simulink model "HANcoder_E407_TTA_Controller_v4_7"  (R2018b)
settings: Solver=FixedStepDiscrete  StartTime=0.0  StopTime=1  FixedStep=0.01  RelTol=1e-3
PreLoadFcn:
  | librarySetup
  | eval([bdroot,'_startup']) %Calling [modelName]_startup.m
values from neighbouring files (symbols this model uses):
  Backup_Board = 0    [HANcoder_E407_TTA_Controller_v3_5_startup.m]    (also in HANcoder_E407_TTA_Controller_v4_6_startup.m; HANcoder_E407_TTA_Controller_v4_7_startup.m; HANcoder_E407_TTA_Controller_v4_startup.m)
  basic_cycle_duration_bc0 = TM_Reset_Board   + COMP_duration    (= 212)    [HANcoder_E407_TTA_Controller_v3_5_startup.m]    (also in HANcoder_E407_TTA_Controller_v4_6_startup.m; HANcoder_E407_TTA_Controller_v4_7_startup.m; HANcoder_E407_TTA_Controller_v4_startup.m)
  basic_cycle_duration_bc1 = TM_Reset_Var_bc1 + COMP_duration    (= 288)    [HANcoder_E407_TTA_Controller_v3_5_startup.m]    (also in HANcoder_E407_TTA_Controller_v4_6_startup.m = 332; HANcoder_E407_TTA_Controller_v4_7_startup.m = 372; HANcoder_E407_TTA_Controller_v4_startup.m = 332)
  comm_delay_estimation1 = round(comm_delay_measured1*hardware_granularity/frequency_IRQ)    [HANcoder_E407_TTA_Controller_v3_5_startup.m]    (also in HANcoder_E407_TTA_Controller_v4_6_startup.m; HANcoder_E407_TTA_Controller_v4_7_startup.m; HANcoder_E407_TTA_Controller_v4_startup.m)
  comm_delay_estimation2 = round(comm_delay_measured2*hardware_granularity/frequency_IRQ)    [HANcoder_E407_TTA_Controller_v3_5_startup.m]    (also in HANcoder_E407_TTA_Controller_v4_6_startup.m; HANcoder_E407_TTA_Controller_v4_7_startup.m; HANcoder_E407_TTA_Controller_v4_startup.m)
  COMM_Period = 40    [HANcoder_E407_TTA_Controller_v3_5_startup.m]    (also in HANcoder_E407_TTA_Controller_v4_6_startup.m; HANcoder_E407_TTA_Controller_v4_7_startup.m; HANcoder_E407_TTA_Controller_v4_startup.m)
  COMM_Phase1 = Simulink.Parameter    [HANcoder_E407_TTA_Controller_v3_5_startup.m]    (also in HANcoder_E407_TTA_Controller_v4_6_startup.m; HANcoder_E407_TTA_Controller_v4_7_startup.m; HANcoder_E407_TTA_Controller_v4_startup.m)
  COMM_Phase2 = Simulink.Parameter    [HANcoder_E407_TTA_Controller_v3_5_startup.m]    (also in HANcoder_E407_TTA_Controller_v4_6_startup.m; HANcoder_E407_TTA_Controller_v4_7_startup.m; HANcoder_E407_TTA_Controller_v4_startup.m)
  COMM_Phase_init1 = Simulink.Parameter    [HANcoder_E407_TTA_Controller_v3_5_startup.m]    (also in HANcoder_E407_TTA_Controller_v4_6_startup.m; HANcoder_E407_TTA_Controller_v4_7_startup.m; HANcoder_E407_TTA_Controller_v4_startup.m)
  COMM_Phase_init2 = Simulink.Parameter    [HANcoder_E407_TTA_Controller_v3_5_startup.m]    (also in HANcoder_E407_TTA_Controller_v4_6_startup.m; HANcoder_E407_TTA_Controller_v4_7_startup.m; HANcoder_E407_TTA_Controller_v4_startup.m)
  COMP_duration = 4    [HANcoder_E407_TTA_Controller_v3_5_startup.m]    (also in HANcoder_E407_TTA_Controller_v4_6_startup.m; HANcoder_E407_TTA_Controller_v4_7_startup.m; HANcoder_E407_TTA_Controller_v4_startup.m)
  Controller1_Board = 1    [HANcoder_E407_TTA_Controller_v3_5_startup.m]    (also in HANcoder_E407_TTA_Controller_v4_6_startup.m; HANcoder_E407_TTA_Controller_v4_7_startup.m; HANcoder_E407_TTA_Controller_v4_startup.m)
  Controller2_Board = 2    [HANcoder_E407_TTA_Controller_v3_5_startup.m]    (also in HANcoder_E407_TTA_Controller_v4_6_startup.m; HANcoder_E407_TTA_Controller_v4_7_startup.m; HANcoder_E407_TTA_Controller_v4_startup.m)
  Controller3_Board = 3    [HANcoder_E407_TTA_Controller_v3_5_startup.m]    (also in HANcoder_E407_TTA_Controller_v4_6_startup.m; HANcoder_E407_TTA_Controller_v4_7_startup.m; HANcoder_E407_TTA_Controller_v4_startup.m)
  delta_a_set = Simulink.Parameter    [HANcoder_E407_TTA_Controller_v3_5_startup.m]    (also in HANcoder_E407_TTA_Controller_v4_6_startup.m; HANcoder_E407_TTA_Controller_v4_7_startup.m; HANcoder_E407_TTA_Controller_v4_startup.m)
  delta_f_set = Simulink.Parameter    [HANcoder_E407_TTA_Controller_v3_5_startup.m]    (also in HANcoder_E407_TTA_Controller_v4_6_startup.m; HANcoder_E407_TTA_Controller_v4_7_startup.m; HANcoder_E407_TTA_Controller_v4_startup.m)
  delta_max = 1    [HANcoder_E407_TTA_Controller_v3_5_startup.m]    (also in HANcoder_E407_TTA_Controller_v4_6_startup.m; HANcoder_E407_TTA_Controller_v4_7_startup.m; HANcoder_E407_TTA_Controller_v4_startup.m)
  delta_min = -1    [HANcoder_E407_TTA_Controller_v3_5_startup.m]    (also in HANcoder_E407_TTA_Controller_v4_6_startup.m; HANcoder_E407_TTA_Controller_v4_7_startup.m; HANcoder_E407_TTA_Controller_v4_startup.m)
  delta_precision = 6    [HANcoder_E407_TTA_Controller_v3_5_startup.m]    (also in HANcoder_E407_TTA_Controller_v4_6_startup.m; HANcoder_E407_TTA_Controller_v4_7_startup.m; HANcoder_E407_TTA_Controller_v4_startup.m)
  e_width = 0.1    [HANcoder_E407_TTA_Controller_v3_5_startup.m]    (also in HANcoder_E407_TTA_Controller_v4_6_startup.m; HANcoder_E407_TTA_Controller_v4_7_startup.m; HANcoder_E407_TTA_Controller_v4_startup.m)
  frequency_IRQ = 100    [HANcoder_E407_2xCAN_TEST_startup.m]    (also in HANcoder_E407_TTA_Controller_v3_5_startup.m; HANcoder_E407_TTA_Controller_v4_6_startup.m; HANcoder_E407_TTA_Controller_v4_7_startup.m; HANcoder_E407_TTA_Controller_v4_startup.m)
  HANtuneOverride = Simulink.Parameter    [HANcoder_E407_2xCAN_TEST_startup.m]    (also in HANcoder_E407_TTA_Controller_v3_5_startup.m; HANcoder_E407_TTA_Controller_v4_6_startup.m; HANcoder_E407_TTA_Controller_v4_7_startup.m; HANcoder_E407_TTA_Controller_v4_startup.m)
  hardware_granularity = 1000000    [HANcoder_E407_2xCAN_TEST_startup.m]    (also in HANcoder_E407_TTA_Controller_v3_5_startup.m; HANcoder_E407_TTA_Controller_v4_6_startup.m; HANcoder_E407_TTA_Controller_v4_7_startup.m; HANcoder_E407_TTA_Controller_v4_startup.m)
  I_a = 2.25    [HANcoder_E407_TTA_Controller_v3_5_startup.m]    (also in HANcoder_E407_TTA_Controller_v4_6_startup.m; HANcoder_E407_TTA_Controller_v4_7_startup.m; HANcoder_E407_TTA_Controller_v4_startup.m)
  I_f = 2.25    [HANcoder_E407_TTA_Controller_v3_5_startup.m]    (also in HANcoder_E407_TTA_Controller_v4_6_startup.m; HANcoder_E407_TTA_Controller_v4_7_startup.m; HANcoder_E407_TTA_Controller_v4_startup.m)
  idle_time_init = basic_cycle_duration_bc0 + basic_cycle_duration_bc1    (= 500)    [HANcoder_E407_TTA_Controller_v3_5_startup.m]    (also in HANcoder_E407_TTA_Controller_v4_6_startup.m = 544; HANcoder_E407_TTA_Controller_v4_7_startup.m = 584; HANcoder_E407_TTA_Controller_v4_startup.m = 544)
  Input_Gen_Board = 4    [HANcoder_E407_TTA_Controller_v3_5_startup.m]    (also in HANcoder_E407_TTA_Controller_v4_6_startup.m; HANcoder_E407_TTA_Controller_v4_7_startup.m; HANcoder_E407_TTA_Controller_v4_startup.m)
  LA_Clock_Gr = 1    [HANcoder_E407_TTA_Controller_v3_5_startup.m]    (also in HANcoder_E407_TTA_Controller_v4_6_startup.m; HANcoder_E407_TTA_Controller_v4_7_startup.m; HANcoder_E407_TTA_Controller_v4_startup.m)
  LA_COMM_dly = 1    [HANcoder_E407_TTA_Controller_v3_5_startup.m]    (also in HANcoder_E407_TTA_Controller_v4_6_startup.m; HANcoder_E407_TTA_Controller_v4_7_startup.m; HANcoder_E407_TTA_Controller_v4_startup.m)
  LA_COMM_Err = 1    [HANcoder_E407_TTA_Controller_v3_5_startup.m]    (also in HANcoder_E407_TTA_Controller_v4_6_startup.m; HANcoder_E407_TTA_Controller_v4_7_startup.m; HANcoder_E407_TTA_Controller_v4_startup.m)
  LA_E_Desync = 1    [HANcoder_E407_TTA_Controller_v3_5_startup.m]    (also in HANcoder_E407_TTA_Controller_v4_6_startup.m; HANcoder_E407_TTA_Controller_v4_7_startup.m; HANcoder_E407_TTA_Controller_v4_startup.m)
  LA_MEX_Flag = 1    [HANcoder_E407_TTA_Controller_v3_5_startup.m]    (also in HANcoder_E407_TTA_Controller_v4_6_startup.m; HANcoder_E407_TTA_Controller_v4_7_startup.m; HANcoder_E407_TTA_Controller_v4_startup.m)
  LA_Task_Act = 1    [HANcoder_E407_TTA_Controller_v3_5_startup.m]    (also in HANcoder_E407_TTA_Controller_v4_6_startup.m; HANcoder_E407_TTA_Controller_v4_7_startup.m; HANcoder_E407_TTA_Controller_v4_startup.m)
  m_v = 100.0    (= 100)    [HANcoder_E407_TTA_Controller_v3_5_startup.m]    (also in HANcoder_E407_TTA_Controller_v4_6_startup.m; HANcoder_E407_TTA_Controller_v4_7_startup.m; HANcoder_E407_TTA_Controller_v4_startup.m)
  Master_Role = 1    [HANcoder_E407_TTA_Controller_v3_5_startup.m]    (also in HANcoder_E407_TTA_Controller_v4_6_startup.m; HANcoder_E407_TTA_Controller_v4_7_startup.m; HANcoder_E407_TTA_Controller_v4_startup.m)
  matrix_cycle_duration = basic_cycle_duration_bc0 + basic_cycle_duration_bc1    (= 500)    [HANcoder_E407_TTA_Controller_v3_5_startup.m]    (also in HANcoder_E407_TTA_Controller_v4_6_startup.m = 544; HANcoder_E407_TTA_Controller_v4_7_startup.m = 584; HANcoder_E407_TTA_Controller_v4_startup.m = 544)
  matrix_rows = 2    [HANcoder_E407_TTA_Controller_v3_5_startup.m]    (also in HANcoder_E407_TTA_Controller_v4_6_startup.m; HANcoder_E407_TTA_Controller_v4_7_startup.m; HANcoder_E407_TTA_Controller_v4_startup.m)
  max_desync = 15    [HANcoder_E407_TTA_Controller_v3_5_startup.m]    (also in HANcoder_E407_TTA_Controller_v4_6_startup.m; HANcoder_E407_TTA_Controller_v4_7_startup.m = 30; HANcoder_E407_TTA_Controller_v4_startup.m)
  max_num_msgs_CAN1 = 2^Tx_bit_number-1    (= 7)    [HANcoder_E407_TTA_Controller_v3_5_startup.m]    (also in HANcoder_E407_TTA_Controller_v4_6_startup.m = 15; HANcoder_E407_TTA_Controller_v4_7_startup.m = 15; HANcoder_E407_TTA_Controller_v4_startup.m)
  max_num_msgs_CAN2 = max_num_msgs_CAN1    (= 7)    [HANcoder_E407_TTA_Controller_v3_5_startup.m]    (also in HANcoder_E407_TTA_Controller_v4_6_startup.m = 15; HANcoder_E407_TTA_Controller_v4_7_startup.m = 15; HANcoder_E407_TTA_Controller_v4_startup.m)
  min_desync = (-1)*max_desync    (= -15)    [HANcoder_E407_TTA_Controller_v3_5_startup.m]    (also in HANcoder_E407_TTA_Controller_v4_6_startup.m; HANcoder_E407_TTA_Controller_v4_7_startup.m = -30; HANcoder_E407_TTA_Controller_v4_startup.m)
  OutControl1_ID = 23    [HANcoder_E407_TTA_Controller_v3_5_startup.m]    (also in HANcoder_E407_TTA_Controller_v4_6_startup.m; HANcoder_E407_TTA_Controller_v4_7_startup.m; HANcoder_E407_TTA_Controller_v4_startup.m)
  OutControl2_ID = 24    [HANcoder_E407_TTA_Controller_v3_5_startup.m]    (also in HANcoder_E407_TTA_Controller_v4_6_startup.m; HANcoder_E407_TTA_Controller_v4_7_startup.m; HANcoder_E407_TTA_Controller_v4_startup.m)
  OutEmulator_ID = 25    [HANcoder_E407_TTA_Controller_v3_5_startup.m]    (also in HANcoder_E407_TTA_Controller_v4_6_startup.m = 26; HANcoder_E407_TTA_Controller_v4_7_startup.m = 26; HANcoder_E407_TTA_Controller_v4_startup.m)
  OutMaster_ID = 25    [HANcoder_E407_TTA_Controller_v4_6_startup.m]    (also in HANcoder_E407_TTA_Controller_v4_7_startup.m; HANcoder_E407_TTA_Controller_v4_startup.m = 26)
  R_al = 0.10    (= 0.1)    [HANcoder_E407_TTA_Controller_v3_5_startup.m]    (also in HANcoder_E407_TTA_Controller_v4_6_startup.m; HANcoder_E407_TTA_Controller_v4_7_startup.m; HANcoder_E407_TTA_Controller_v4_startup.m)
  R_ar = 0.10    (= 0.1)    [HANcoder_E407_TTA_Controller_v3_5_startup.m]    (also in HANcoder_E407_TTA_Controller_v4_6_startup.m; HANcoder_E407_TTA_Controller_v4_7_startup.m; HANcoder_E407_TTA_Controller_v4_startup.m)
  R_fl = 0.10    (= 0.1)    [HANcoder_E407_TTA_Controller_v3_5_startup.m]    (also in HANcoder_E407_TTA_Controller_v4_6_startup.m; HANcoder_E407_TTA_Controller_v4_7_startup.m; HANcoder_E407_TTA_Controller_v4_startup.m)
  R_fr = 0.10    (= 0.1)    [HANcoder_E407_TTA_Controller_v3_5_startup.m]    (also in HANcoder_E407_TTA_Controller_v4_6_startup.m; HANcoder_E407_TTA_Controller_v4_7_startup.m; HANcoder_E407_TTA_Controller_v4_startup.m)
  script_run = Simulink.Parameter    [HANcoder_E407_TTA_Controller_v3_5_startup.m]    (also in HANcoder_E407_TTA_Controller_v4_6_startup.m; HANcoder_E407_TTA_Controller_v4_7_startup.m; HANcoder_E407_TTA_Controller_v4_startup.m)
  SensorValues_ID = 22    [HANcoder_E407_TTA_Controller_v3_5_startup.m]    (also in HANcoder_E407_TTA_Controller_v4_6_startup.m; HANcoder_E407_TTA_Controller_v4_7_startup.m; HANcoder_E407_TTA_Controller_v4_startup.m)
  SetValues_ID = 21    [HANcoder_E407_TTA_Controller_v3_5_startup.m]    (also in HANcoder_E407_TTA_Controller_v4_6_startup.m; HANcoder_E407_TTA_Controller_v4_7_startup.m; HANcoder_E407_TTA_Controller_v4_startup.m)
  Slave_Role = 2    [HANcoder_E407_TTA_Controller_v3_5_startup.m]    (also in HANcoder_E407_TTA_Controller_v4_6_startup.m; HANcoder_E407_TTA_Controller_v4_7_startup.m; HANcoder_E407_TTA_Controller_v4_startup.m)
  speed_k_d = Simulink.Parameter    [HANcoder_E407_TTA_Controller_v3_5_startup.m]    (also in HANcoder_E407_TTA_Controller_v4_6_startup.m; HANcoder_E407_TTA_Controller_v4_7_startup.m; HANcoder_E407_TTA_Controller_v4_startup.m)
  speed_k_i = Simulink.Parameter    [HANcoder_E407_TTA_Controller_v3_5_startup.m]    (also in HANcoder_E407_TTA_Controller_v4_6_startup.m; HANcoder_E407_TTA_Controller_v4_7_startup.m; HANcoder_E407_TTA_Controller_v4_startup.m)
  speed_k_p = Simulink.Parameter    [HANcoder_E407_TTA_Controller_v3_5_startup.m]    (also in HANcoder_E407_TTA_Controller_v4_6_startup.m; HANcoder_E407_TTA_Controller_v4_7_startup.m; HANcoder_E407_TTA_Controller_v4_startup.m)
  speed_max = 10    [HANcoder_E407_TTA_Controller_v3_5_startup.m]    (also in HANcoder_E407_TTA_Controller_v4_6_startup.m; HANcoder_E407_TTA_Controller_v4_7_startup.m; HANcoder_E407_TTA_Controller_v4_startup.m)
  speed_min = -10    [HANcoder_E407_TTA_Controller_v3_5_startup.m]    (also in HANcoder_E407_TTA_Controller_v4_6_startup.m; HANcoder_E407_TTA_Controller_v4_7_startup.m; HANcoder_E407_TTA_Controller_v4_startup.m)
  speed_precision = 3    [HANcoder_E407_TTA_Controller_v3_5_startup.m]    (also in HANcoder_E407_TTA_Controller_v4_6_startup.m; HANcoder_E407_TTA_Controller_v4_7_startup.m; HANcoder_E407_TTA_Controller_v4_startup.m)
  Sync_ID = 1    [HANcoder_E407_TTA_Controller_v3_5_startup.m]    (also in HANcoder_E407_TTA_Controller_v4_6_startup.m; HANcoder_E407_TTA_Controller_v4_7_startup.m; HANcoder_E407_TTA_Controller_v4_startup.m)
  tau_max = 5    [HANcoder_E407_TTA_Controller_v3_5_startup.m]    (also in HANcoder_E407_TTA_Controller_v4_6_startup.m; HANcoder_E407_TTA_Controller_v4_7_startup.m; HANcoder_E407_TTA_Controller_v4_startup.m)
  tau_min = -5    [HANcoder_E407_TTA_Controller_v3_5_startup.m]    (also in HANcoder_E407_TTA_Controller_v4_6_startup.m; HANcoder_E407_TTA_Controller_v4_7_startup.m; HANcoder_E407_TTA_Controller_v4_startup.m)
  tau_range = abs(tau_max) + abs(tau_min)    [HANcoder_E407_TTA_Controller_v3_5_startup.m]    (also in HANcoder_E407_TTA_Controller_v4_6_startup.m; HANcoder_E407_TTA_Controller_v4_7_startup.m; HANcoder_E407_TTA_Controller_v4_startup.m)
  theta_max = (speed_max/R_fr)*matrix_cycle_duration*frequency_IRQ/hardware_granularity    (= 5)    [HANcoder_E407_TTA_Controller_v3_5_startup.m]    (also in HANcoder_E407_TTA_Controller_v4_6_startup.m = 5.44; HANcoder_E407_TTA_Controller_v4_7_startup.m = 5.84; HANcoder_E407_TTA_Controller_v4_startup.m = 5.44)
  theta_min = (-1)*theta_max    (= -5)    [HANcoder_E407_TTA_Controller_v3_5_startup.m]    (also in HANcoder_E407_TTA_Controller_v4_6_startup.m = -5.44; HANcoder_E407_TTA_Controller_v4_7_startup.m = -5.84; HANcoder_E407_TTA_Controller_v4_startup.m = -5.44)
  theta_precision = 7-(fix(log2(theta_max))+1)    [HANcoder_E407_TTA_Controller_v3_5_startup.m]    (also in HANcoder_E407_TTA_Controller_v4_6_startup.m; HANcoder_E407_TTA_Controller_v4_7_startup.m; HANcoder_E407_TTA_Controller_v4_startup.m)
  Tl_a = 0.6    [HANcoder_E407_TTA_Controller_v3_5_startup.m]    (also in HANcoder_E407_TTA_Controller_v4_6_startup.m; HANcoder_E407_TTA_Controller_v4_7_startup.m; HANcoder_E407_TTA_Controller_v4_startup.m)
  Tl_f = 0.6    [HANcoder_E407_TTA_Controller_v3_5_startup.m]    (also in HANcoder_E407_TTA_Controller_v4_6_startup.m; HANcoder_E407_TTA_Controller_v4_7_startup.m; HANcoder_E407_TTA_Controller_v4_startup.m)
  TM_Check_Output_Control1 = TM_COMM_Output_Control1 + COMM_duration    (= 188)    [HANcoder_E407_TTA_Controller_v3_5_startup.m]    (also in HANcoder_E407_TTA_Controller_v4_6_startup.m; HANcoder_E407_TTA_Controller_v4_7_startup.m; HANcoder_E407_TTA_Controller_v4_startup.m)
  TM_Check_Output_Control2 = TM_COMM_Output_Control2 + COMM_duration    (= 232)    [HANcoder_E407_TTA_Controller_v3_5_startup.m]    (also in HANcoder_E407_TTA_Controller_v4_6_startup.m; HANcoder_E407_TTA_Controller_v4_7_startup.m; HANcoder_E407_TTA_Controller_v4_startup.m)
  TM_Check_Output_Emulator = TM_COMM_Output_Emulator + COMM_duration    (= 280)    [HANcoder_E407_TTA_Controller_v3_5_startup.m]    (also in HANcoder_E407_TTA_Controller_v4_6_startup.m = 320; HANcoder_E407_TTA_Controller_v4_7_startup.m = 360; HANcoder_E407_TTA_Controller_v4_startup.m = 320)
  TM_Check_Output_Emulator_2 = TM_Check_Output_Emulator + 2    (= 282)    [HANcoder_E407_TTA_Controller_v3_5_startup.m]    (also in HANcoder_E407_TTA_Controller_v4_6_startup.m = 322; HANcoder_E407_TTA_Controller_v4_7_startup.m = 362; HANcoder_E407_TTA_Controller_v4_startup.m = 322)
  TM_Check_Output_Emulator_3 = TM_Check_Output_Emulator_2 + 2    (= 324)    [HANcoder_E407_TTA_Controller_v4_6_startup.m]    (also in HANcoder_E407_TTA_Controller_v4_7_startup.m = 364; HANcoder_E407_TTA_Controller_v4_startup.m)
  TM_Check_Output_Master = TM_COMM_Output_Master + COMM_duration    (= 312)    [HANcoder_E407_TTA_Controller_v4_7_startup.m]
  TM_Check_Sensor_Values = TM_COMM_Sensor_Values + COMM_duration    (= 132)    [HANcoder_E407_TTA_Controller_v3_5_startup.m]    (also in HANcoder_E407_TTA_Controller_v4_6_startup.m; HANcoder_E407_TTA_Controller_v4_7_startup.m; HANcoder_E407_TTA_Controller_v4_startup.m)
  TM_Check_Sensor_Values_2 = TM_Check_Sensor_Values + 2    (= 134)    [HANcoder_E407_TTA_Controller_v3_5_startup.m]    (also in HANcoder_E407_TTA_Controller_v4_6_startup.m; HANcoder_E407_TTA_Controller_v4_7_startup.m; HANcoder_E407_TTA_Controller_v4_startup.m)
  TM_Check_Set_Values = TM_COMM_Set_Values + COMM_duration    (= 88)    [HANcoder_E407_TTA_Controller_v3_5_startup.m]    (also in HANcoder_E407_TTA_Controller_v4_6_startup.m; HANcoder_E407_TTA_Controller_v4_7_startup.m; HANcoder_E407_TTA_Controller_v4_startup.m)
  TM_Check_Set_Values_2 = TM_Check_Set_Values + 2    (= 90)    [HANcoder_E407_TTA_Controller_v3_5_startup.m]    (also in HANcoder_E407_TTA_Controller_v4_6_startup.m; HANcoder_E407_TTA_Controller_v4_7_startup.m; HANcoder_E407_TTA_Controller_v4_startup.m)
  TM_Check_Sync = TM_COMM_Sync   + COMM_duration    (= 40)    [HANcoder_E407_TTA_Controller_v3_5_startup.m]    (also in HANcoder_E407_TTA_Controller_v4_6_startup.m; HANcoder_E407_TTA_Controller_v4_7_startup.m; HANcoder_E407_TTA_Controller_v4_startup.m)
  TM_Check_TOuts = TM_Count_Vote3 + COMP_duration    (= 196)    [HANcoder_E407_TTA_Controller_v3_5_startup.m]    (also in HANcoder_E407_TTA_Controller_v4_6_startup.m; HANcoder_E407_TTA_Controller_v4_7_startup.m; HANcoder_E407_TTA_Controller_v4_startup.m)
  TM_Check_Vote1 = TM_COMM_Vote1  + COMM_duration    (= 92)    [HANcoder_E407_TTA_Controller_v3_5_startup.m]    (also in HANcoder_E407_TTA_Controller_v4_6_startup.m; HANcoder_E407_TTA_Controller_v4_7_startup.m; HANcoder_E407_TTA_Controller_v4_startup.m)
  TM_Check_Vote2 = TM_COMM_Vote2  + COMM_duration    (= 140)    [HANcoder_E407_TTA_Controller_v3_5_startup.m]    (also in HANcoder_E407_TTA_Controller_v4_6_startup.m; HANcoder_E407_TTA_Controller_v4_7_startup.m; HANcoder_E407_TTA_Controller_v4_startup.m)
  TM_Check_Vote2_2 = TM_Check_Vote2 + 2    (= 142)    [HANcoder_E407_TTA_Controller_v3_5_startup.m]    (also in HANcoder_E407_TTA_Controller_v4_6_startup.m; HANcoder_E407_TTA_Controller_v4_7_startup.m; HANcoder_E407_TTA_Controller_v4_startup.m)
  TM_Check_Vote3 = TM_COMM_Vote3  + COMM_duration    (= 188)    [HANcoder_E407_TTA_Controller_v3_5_startup.m]    (also in HANcoder_E407_TTA_Controller_v4_6_startup.m; HANcoder_E407_TTA_Controller_v4_7_startup.m; HANcoder_E407_TTA_Controller_v4_startup.m)
  TM_COMM_Output_Control1 = TM_Velocity + COMP_duration    (= 148)    [HANcoder_E407_TTA_Controller_v3_5_startup.m]    (also in HANcoder_E407_TTA_Controller_v4_6_startup.m; HANcoder_E407_TTA_Controller_v4_7_startup.m; HANcoder_E407_TTA_Controller_v4_startup.m)
  TM_COMM_Output_Control2 = TM_Check_Output_Control1 + COMP_duration    (= 192)    [HANcoder_E407_TTA_Controller_v3_5_startup.m]    (also in HANcoder_E407_TTA_Controller_v4_6_startup.m; HANcoder_E407_TTA_Controller_v4_7_startup.m; HANcoder_E407_TTA_Controller_v4_startup.m)
  TM_COMM_Output_Emulator = TM_TMR + COMP_duration    (= 240)    [HANcoder_E407_TTA_Controller_v3_5_startup.m]    (also in HANcoder_E407_TTA_Controller_v4_6_startup.m = 280; HANcoder_E407_TTA_Controller_v4_7_startup.m = 320; HANcoder_E407_TTA_Controller_v4_startup.m = 280)
  TM_COMM_Output_Master = TM_Check_Output_Control2 + COMM_duration    (= 272)    [HANcoder_E407_TTA_Controller_v4_6_startup.m]    (also in HANcoder_E407_TTA_Controller_v4_7_startup.m; HANcoder_E407_TTA_Controller_v4_startup.m)
  TM_COMM_Sensor_Values = TM_Check_Set_Values + COMP_duration    (= 92)    [HANcoder_E407_TTA_Controller_v3_5_startup.m]    (also in HANcoder_E407_TTA_Controller_v4_6_startup.m; HANcoder_E407_TTA_Controller_v4_7_startup.m; HANcoder_E407_TTA_Controller_v4_startup.m)
  TM_COMM_Set_Values = TM_Update_LT + COMP_duration    (= 48)    [HANcoder_E407_TTA_Controller_v3_5_startup.m]    (also in HANcoder_E407_TTA_Controller_v4_6_startup.m; HANcoder_E407_TTA_Controller_v4_7_startup.m; HANcoder_E407_TTA_Controller_v4_startup.m)
  TM_COMM_Sync = basic_cycle_start    (= 0)    [HANcoder_E407_TTA_Controller_v3_5_startup.m]    (also in HANcoder_E407_TTA_Controller_v4_6_startup.m; HANcoder_E407_TTA_Controller_v4_7_startup.m; HANcoder_E407_TTA_Controller_v4_startup.m)
  TM_COMM_Vote1 = TM_Vote_Dec    + COMP_duration    (= 52)    [HANcoder_E407_TTA_Controller_v3_5_startup.m]    (also in HANcoder_E407_TTA_Controller_v4_6_startup.m; HANcoder_E407_TTA_Controller_v4_7_startup.m; HANcoder_E407_TTA_Controller_v4_startup.m)
  TM_COMM_Vote2 = TM_Count_Vote1 + COMP_duration    (= 100)    [HANcoder_E407_TTA_Controller_v3_5_startup.m]    (also in HANcoder_E407_TTA_Controller_v4_6_startup.m; HANcoder_E407_TTA_Controller_v4_7_startup.m; HANcoder_E407_TTA_Controller_v4_startup.m)
  TM_COMM_Vote3 = TM_Count_Vote2 + COMP_duration    (= 148)    [HANcoder_E407_TTA_Controller_v3_5_startup.m]    (also in HANcoder_E407_TTA_Controller_v4_6_startup.m; HANcoder_E407_TTA_Controller_v4_7_startup.m; HANcoder_E407_TTA_Controller_v4_startup.m)
  TM_Count_Vote1 = TM_Check_Vote1 + COMP_duration    (= 96)    [HANcoder_E407_TTA_Controller_v3_5_startup.m]    (also in HANcoder_E407_TTA_Controller_v4_6_startup.m; HANcoder_E407_TTA_Controller_v4_7_startup.m; HANcoder_E407_TTA_Controller_v4_startup.m)
  TM_Count_Vote2 = TM_Check_Vote2 + COMP_duration    (= 144)    [HANcoder_E407_TTA_Controller_v3_5_startup.m]    (also in HANcoder_E407_TTA_Controller_v4_6_startup.m; HANcoder_E407_TTA_Controller_v4_7_startup.m; HANcoder_E407_TTA_Controller_v4_startup.m)
  TM_Count_Vote3 = TM_Check_Vote3 + COMP_duration    (= 192)    [HANcoder_E407_TTA_Controller_v3_5_startup.m]    (also in HANcoder_E407_TTA_Controller_v4_6_startup.m; HANcoder_E407_TTA_Controller_v4_7_startup.m; HANcoder_E407_TTA_Controller_v4_startup.m)
  TM_Data_bc0 = TM_COMM_Sync    (= 0)    [HANcoder_E407_TTA_Controller_v3_5_startup.m]    (also in HANcoder_E407_TTA_Controller_v4_6_startup.m; HANcoder_E407_TTA_Controller_v4_7_startup.m; HANcoder_E407_TTA_Controller_v4_startup.m)
  TM_Data_bc1 = TM_Data_bc0(1:4)    [HANcoder_E407_TTA_Controller_v3_5_startup.m]    (also in HANcoder_E407_TTA_Controller_v4_6_startup.m; HANcoder_E407_TTA_Controller_v4_7_startup.m; HANcoder_E407_TTA_Controller_v4_startup.m)
  TM_New_Master = TM_Check_TOuts + COMP_duration    (= 200)    [HANcoder_E407_TTA_Controller_v3_5_startup.m]    (also in HANcoder_E407_TTA_Controller_v4_6_startup.m; HANcoder_E407_TTA_Controller_v4_7_startup.m; HANcoder_E407_TTA_Controller_v4_startup.m)
  TM_Reset_Board = TM_Reset_Var   + COMP_duration    (= 208)    [HANcoder_E407_TTA_Controller_v3_5_startup.m]    (also in HANcoder_E407_TTA_Controller_v4_6_startup.m; HANcoder_E407_TTA_Controller_v4_7_startup.m; HANcoder_E407_TTA_Controller_v4_startup.m)
  TM_Reset_Var = TM_New_Master  + COMP_duration    (= 204)    [HANcoder_E407_TTA_Controller_v3_5_startup.m]    (also in HANcoder_E407_TTA_Controller_v4_6_startup.m; HANcoder_E407_TTA_Controller_v4_7_startup.m; HANcoder_E407_TTA_Controller_v4_startup.m)
  TM_Reset_Var_bc1 = TM_Check_Output_Emulator + COMP_duration    (= 284)    [HANcoder_E407_TTA_Controller_v3_5_startup.m]    (also in HANcoder_E407_TTA_Controller_v4_6_startup.m = 328; HANcoder_E407_TTA_Controller_v4_7_startup.m = 368; HANcoder_E407_TTA_Controller_v4_startup.m = 328)
  TM_Reset_Var_bc1_2 = TM_Reset_Var_bc1 + 2    (= 286)    [HANcoder_E407_TTA_Controller_v3_5_startup.m]    (also in HANcoder_E407_TTA_Controller_v4_6_startup.m = 330; HANcoder_E407_TTA_Controller_v4_7_startup.m = 370; HANcoder_E407_TTA_Controller_v4_startup.m = 330)
  TM_Steer = TM_Check_Sensor_Values + COMP_duration    (= 136)    [HANcoder_E407_TTA_Controller_v3_5_startup.m]    (also in HANcoder_E407_TTA_Controller_v4_6_startup.m; HANcoder_E407_TTA_Controller_v4_7_startup.m; HANcoder_E407_TTA_Controller_v4_startup.m)
  TM_TMR = TM_Check_Output_Control2 + COMP_duration    (= 236)    [HANcoder_E407_TTA_Controller_v3_5_startup.m]    (also in HANcoder_E407_TTA_Controller_v4_6_startup.m = 276; HANcoder_E407_TTA_Controller_v4_7_startup.m = 316; HANcoder_E407_TTA_Controller_v4_startup.m = 276)
  TM_TMR_2 = TM_TMR + 1    (= 237)    [HANcoder_E407_TTA_Controller_v3_5_startup.m]    (also in HANcoder_E407_TTA_Controller_v4_6_startup.m = 277; HANcoder_E407_TTA_Controller_v4_7_startup.m = 317; HANcoder_E407_TTA_Controller_v4_startup.m = 277)
  TM_TMR_3 = TM_TMR + 3    (= 239)    [HANcoder_E407_TTA_Controller_v3_5_startup.m]    (also in HANcoder_E407_TTA_Controller_v4_6_startup.m = 279; HANcoder_E407_TTA_Controller_v4_7_startup.m = 319; HANcoder_E407_TTA_Controller_v4_startup.m = 279)
  TM_Torque = TM_Steer + COMP_duration    (= 140)    [HANcoder_E407_TTA_Controller_v3_5_startup.m]    (also in HANcoder_E407_TTA_Controller_v4_6_startup.m; HANcoder_E407_TTA_Controller_v4_7_startup.m; HANcoder_E407_TTA_Controller_v4_startup.m)
  TM_Type_bc0 = COMM    (= 0)    [HANcoder_E407_TTA_Controller_v3_5_startup.m]    (also in HANcoder_E407_TTA_Controller_v4_6_startup.m; HANcoder_E407_TTA_Controller_v4_7_startup.m; HANcoder_E407_TTA_Controller_v4_startup.m)
  TM_Type_bc1 = TM_Type_bc0(1:4)    [HANcoder_E407_TTA_Controller_v3_5_startup.m]    (also in HANcoder_E407_TTA_Controller_v4_6_startup.m; HANcoder_E407_TTA_Controller_v4_7_startup.m; HANcoder_E407_TTA_Controller_v4_startup.m)
  TM_Update_LT = TM_Check_Sync  + COMP_duration    (= 44)    [HANcoder_E407_TTA_Controller_v3_5_startup.m]    (also in HANcoder_E407_TTA_Controller_v4_6_startup.m; HANcoder_E407_TTA_Controller_v4_7_startup.m; HANcoder_E407_TTA_Controller_v4_startup.m)
  TM_Update_LT_2 = TM_Update_LT   + 2    (= 46)    [HANcoder_E407_TTA_Controller_v3_5_startup.m]    (also in HANcoder_E407_TTA_Controller_v4_6_startup.m; HANcoder_E407_TTA_Controller_v4_7_startup.m; HANcoder_E407_TTA_Controller_v4_startup.m)
  TM_Velocity = TM_Torque + COMP_duration    (= 144)    [HANcoder_E407_TTA_Controller_v3_5_startup.m]    (also in HANcoder_E407_TTA_Controller_v4_6_startup.m; HANcoder_E407_TTA_Controller_v4_7_startup.m; HANcoder_E407_TTA_Controller_v4_startup.m)
  TM_Vote_Dec = TM_Update_LT   + COMP_duration    (= 48)    [HANcoder_E407_TTA_Controller_v3_5_startup.m]    (also in HANcoder_E407_TTA_Controller_v4_6_startup.m; HANcoder_E407_TTA_Controller_v4_7_startup.m; HANcoder_E407_TTA_Controller_v4_startup.m)
  TM_Vote_Dec_2 = TM_Vote_Dec    + 2    (= 50)    [HANcoder_E407_TTA_Controller_v3_5_startup.m]    (also in HANcoder_E407_TTA_Controller_v4_6_startup.m; HANcoder_E407_TTA_Controller_v4_7_startup.m; HANcoder_E407_TTA_Controller_v4_startup.m)
  torque_a_k_d = Simulink.Parameter    [HANcoder_E407_TTA_Controller_v3_5_startup.m]    (also in HANcoder_E407_TTA_Controller_v4_6_startup.m; HANcoder_E407_TTA_Controller_v4_7_startup.m; HANcoder_E407_TTA_Controller_v4_startup.m)
  torque_a_k_i = Simulink.Parameter    [HANcoder_E407_TTA_Controller_v3_5_startup.m]    (also in HANcoder_E407_TTA_Controller_v4_6_startup.m; HANcoder_E407_TTA_Controller_v4_7_startup.m; HANcoder_E407_TTA_Controller_v4_startup.m)
  torque_a_k_p = Simulink.Parameter    [HANcoder_E407_TTA_Controller_v3_5_startup.m]    (also in HANcoder_E407_TTA_Controller_v4_6_startup.m; HANcoder_E407_TTA_Controller_v4_7_startup.m; HANcoder_E407_TTA_Controller_v4_startup.m)
  torque_f_k_d = Simulink.Parameter    [HANcoder_E407_TTA_Controller_v3_5_startup.m]    (also in HANcoder_E407_TTA_Controller_v4_6_startup.m; HANcoder_E407_TTA_Controller_v4_7_startup.m; HANcoder_E407_TTA_Controller_v4_startup.m)
  ... (+8 more)
undefined symbols (not defined in the file or in its folder): A0, A1, A2, A3, A4, CON2, CON3, CON4, D10, D12, D13, D2, D3, D8, D9
libraries: hdlsllib x477, HANcoder_STM32_Target x30, simulink x3, simulink_extras x1
(part 3 of 80)

== system HANcoder_E407_TTA_Controller_v4_7/HANcoder STM32 Target - E407-STM32 algorithm/TTA CAN System/Measure EXecution time ==
  note: Measured Execution Time
  Trigger : TriggerPort  TriggerType=function-call  VariantControl=Variant
  Constant1 : Constant  Priority=1  Value=LA_MEX_Flag
  DEBUG - Toggle digital pin A3 : Subsystem  Priority=3
  Data Store Memory4 : DataStoreMemory  DataStoreName=A3_Pin_State  ReadBeforeWriteMsg=warning  WriteAfterWriteMsg=warning  WriteAfterReadMsg=warning  ShowAdditionalParam=off  OutDataTypeStr=boolean
  wires:
  Constant1/1 -> DEBUG - Toggle digital pin A3/Enable

== system HANcoder_E407_TTA_Controller_v4_7/HANcoder STM32 Target - E407-STM32 algorithm/TTA CAN System/Output Compare Init ==
  S-Function : S-Function  FunctionName=sfcn_timeout_init  SFunctionDeploymentMode=off  EnableBusSupport=off
  Term1 : Terminator
  wires:
  S-Function/1 -> Term1/1

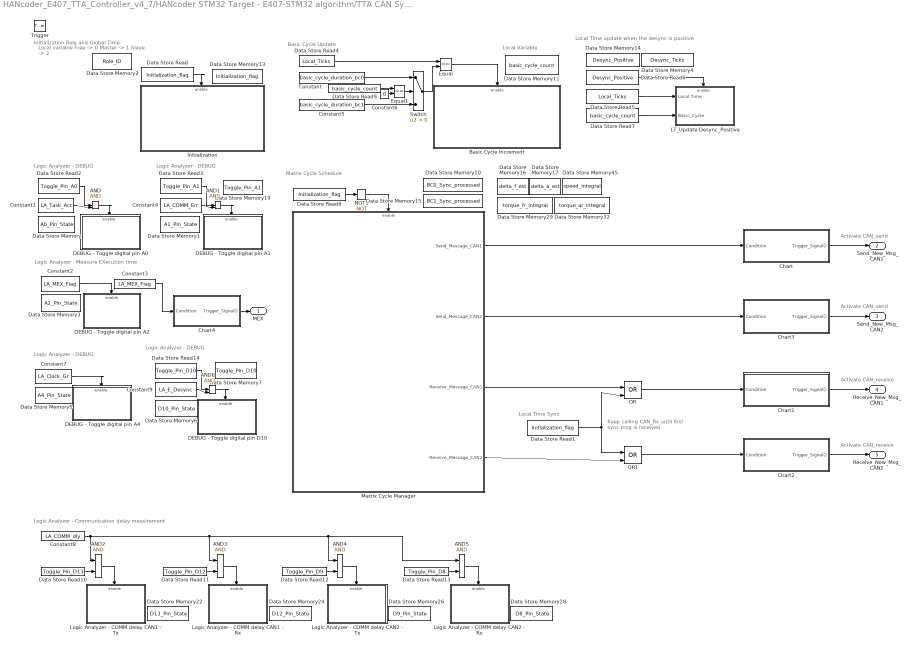
== system HANcoder_E407_TTA_Controller_v4_7/HANcoder STM32 Target - E407-STM32 algorithm/TTA CAN System/TTA System ==
  note: Local Time update when the desync is positive
  note: Logic Analyzer - Measure EXecution time
  note: Keep calling CAN_Rx until
      | first sync msg is received
  note: Logic Analyzer - DEBUG
  note: Local Time Sync
  note: Matrix Cycle Schedule
  note: Initialization Role and Global Time
  note: Activate CAN_send
  note: Basic Cycle Update
  note: Local variable
      |    Free     -> 0
      |    Master -> 1
      |    Slave   -> 2
  note: Local Variable
  note: Activate CAN_receive
  note: Activate CAN_receive
  note: Activate CAN_send
  note: Logic Analyzer - DEBUG
  note: Logic Analyzer - DEBUG
  note: Logic Analyzer - Communication delay measirement
  note: Logic Analyzer - DEBUG
  Trigger : TriggerPort  TriggerType=function-call  VariantControl=Variant  PortDimensions=1
  AND : Logic  Priority=73  IconShape=distinctive  AllPortsSameDT=off  OutDataTypeStr=boolean
  AND1 : Logic  Priority=73  IconShape=distinctive  AllPortsSameDT=off  OutDataTypeStr=boolean
  AND{2..5} (4 alike) : Logic  IconShape=distinctive  AllPortsSameDT=off  OutDataTypeStr=boolean
  AND6 : Logic  Priority=73  IconShape=distinctive  AllPortsSameDT=off  OutDataTypeStr=boolean
  Basic Cycle Increment : Subsystem  Priority=24  TreatAsAtomicUnit=on
  Chart : Stateflow chart  TreatAsAtomicUnit=on
  Chart1 : Stateflow chart  TreatAsAtomicUnit=on
  Chart2 : Stateflow chart  TreatAsAtomicUnit=on
  Chart3 : Stateflow chart  TreatAsAtomicUnit=on
  Chart4 : Stateflow chart  TreatAsAtomicUnit=on
  Constant : Constant  Priority=22  Value=basic_cycle_duration_bc0
  Constant1 : Constant  Priority=72  Value=LA_Task_Act
  Constant2 : Constant  Priority=1  Value=LA_MEX_Flag
  Constant3 : Constant  Priority=100  Value=LA_MEX_Flag
  Constant4 : Constant  Priority=72  Value=LA_COMM_Err
  Constant5 : Constant  Priority=22  Value=basic_cycle_duration_bc1
  Constant6 : Constant  Value=0
  Constant7 : Constant  Priority=72  Value=LA_Clock_Gr
  Constant8 : Constant  Value=LA_COMM_dly
  Constant9 : Constant  Priority=72  Value=LA_E_Desync
  DEBUG - Toggle digital pin A0 : Subsystem  Priority=74
  DEBUG - Toggle digital pin A1 : Subsystem  Priority=74
  DEBUG - Toggle digital pin A2 : Subsystem  Priority=3
  DEBUG - Toggle digital pin A4 : Subsystem  Priority=74
  DEBUG - Toggle digital pin D10 : Subsystem  Priority=74
  Data Store Memory : DataStoreMemory  Priority=70  DataStoreName=A0_Pin_State  ReadBeforeWriteMsg=warning  WriteAfterWriteMsg=warning  WriteAfterReadMsg=warning  ShowAdditionalParam=off  OutDataTypeStr=boolean
  Data Store Memory1 : DataStoreMemory  Priority=70  DataStoreName=A1_Pin_State  ReadBeforeWriteMsg=warning  WriteAfterWriteMsg=warning  WriteAfterReadMsg=warning  ShowAdditionalParam=off  OutDataTypeStr=boolean
  Data Store Memory10 : DataStoreMemory  Priority=30  DataStoreName=BC0_Sync_processed  ReadBeforeWriteMsg=warning  WriteAfterWriteMsg=warning  WriteAfterReadMsg=warning  ShowAdditionalParam=off  OutDataTypeStr=boolean
  Data Store Memory11 : DataStoreMemory  Priority=20  DataStoreName=basic_cycle_count  ReadBeforeWriteMsg=warning  WriteAfterWriteMsg=warning  WriteAfterReadMsg=warning  ShowAdditionalParam=off  OutDataTypeStr=uint8
  Data Store Memory13 : DataStoreMemory  Priority=6  DataStoreName=Initialization_flag  ReadBeforeWriteMsg=warning  WriteAfterWriteMsg=warning  WriteAfterReadMsg=warning  InitialValue=1  ShowAdditionalParam=off  OutDataTypeStr=boolean
  Data Store Memory14 : DataStoreMemory  DataStoreName=Desync_Positive  ReadBeforeWriteMsg=warning  WriteAfterWriteMsg=warning  WriteAfterReadMsg=warning  ShowAdditionalParam=off  OutDataTypeStr=boolean
  Data Store Memory15 : DataStoreMemory  Priority=30  DataStoreName=BC1_Sync_processed  ReadBeforeWriteMsg=warning  WriteAfterWriteMsg=warning  WriteAfterReadMsg=warning  ShowAdditionalParam=off  OutDataTypeStr=boolean
  Data Store Memory16 : DataStoreMemory  DataStoreName=delta_f_est  ReadBeforeWriteMsg=warning  WriteAfterWriteMsg=warning  WriteAfterReadMsg=warning  ShowAdditionalParam=off
  Data Store Memory17 : DataStoreMemory  DataStoreName=delta_a_est  ReadBeforeWriteMsg=warning  WriteAfterWriteMsg=warning  WriteAfterReadMsg=warning  ShowAdditionalParam=off
  Data Store Memory19 : DataStoreMemory  Priority=9  DataStoreName=Toggle_Pin_A1  ReadBeforeWriteMsg=warning  WriteAfterWriteMsg=warning  WriteAfterReadMsg=warning  ShowAdditionalParam=off
  Data Store Memory2 : DataStoreMemory  Priority=5  DataStoreName=Role_ID  ReadBeforeWriteMsg=warning  WriteAfterWriteMsg=warning  WriteAfterReadMsg=warning  ShowAdditionalParam=off
  Data Store Memory22 : DataStoreMemory  Priority=2  DataStoreName=D13_Pin_State  ReadBeforeWriteMsg=warning  WriteAfterWriteMsg=warning  WriteAfterReadMsg=warning  ShowAdditionalParam=off  OutDataTypeStr=boolean
  Data Store Memory24 : DataStoreMemory  Priority=2  DataStoreName=D12_Pin_State  ReadBeforeWriteMsg=warning  WriteAfterWriteMsg=warning  WriteAfterReadMsg=warning  ShowAdditionalParam=off  OutDataTypeStr=boolean
  Data Store Memory26 : DataStoreMemory  Priority=2  DataStoreName=D9_Pin_State  ReadBeforeWriteMsg=warning  WriteAfterWriteMsg=warning  WriteAfterReadMsg=warning  ShowAdditionalParam=off  OutDataTypeStr=boolean
  Data Store Memory28 : DataStoreMemory  Priority=2  DataStoreName=D8_Pin_State  ReadBeforeWriteMsg=warning  WriteAfterWriteMsg=warning  WriteAfterReadMsg=warning  ShowAdditionalParam=off  OutDataTypeStr=boolean
  Data Store Memory29 : DataStoreMemory  DataStoreName=torque_fr_integral  ReadBeforeWriteMsg=warning  WriteAfterWriteMsg=warning  WriteAfterReadMsg=warning  ShowAdditionalParam=off
  Data Store Memory3 : DataStoreMemory  Priority=2  DataStoreName=A2_Pin_State  ReadBeforeWriteMsg=warning  WriteAfterWriteMsg=warning  WriteAfterReadMsg=warning  ShowAdditionalParam=off  OutDataTypeStr=boolean
  Data Store Memory32 : DataStoreMemory  DataStoreName=torque_ar_integral  ReadBeforeWriteMsg=warning  WriteAfterWriteMsg=warning  WriteAfterReadMsg=warning  ShowAdditionalParam=off
  Data Store Memory4 : DataStoreMemory  DataStoreName=Desync_Ticks  ReadBeforeWriteMsg=warning  WriteAfterWriteMsg=warning  WriteAfterReadMsg=warning  ShowAdditionalParam=off
  Data Store Memory45 : DataStoreMemory  DataStoreName=speed_integral  ReadBeforeWriteMsg=warning  WriteAfterWriteMsg=warning  WriteAfterReadMsg=warning  ShowAdditionalParam=off
  Data Store Memory5 : DataStoreMemory  Priority=70  DataStoreName=A4_Pin_State  ReadBeforeWriteMsg=warning  WriteAfterWriteMsg=warning  WriteAfterReadMsg=warning  ShowAdditionalParam=off  OutDataTypeStr=boolean
  Data Store Memory6 : DataStoreMemory  Priority=70  DataStoreName=D10_Pin_State  ReadBeforeWriteMsg=warning  WriteAfterWriteMsg=warning  WriteAfterReadMsg=warning  ShowAdditionalParam=off  OutDataTypeStr=boolean
  Data Store Memory7 : DataStoreMemory  Priority=9  DataStoreName=Toggle_Pin_D10  ReadBeforeWriteMsg=warning  WriteAfterWriteMsg=warning  WriteAfterReadMsg=warning  ShowAdditionalParam=off
  Data Store Read : DataStoreRead  Priority=7  DataStoreName=Initialization_flag
  Data Store Read1 : DataStoreRead  Priority=53  DataStoreName=Initialization_flag
  Data Store Read10 : DataStoreRead  DataStoreName=Toggle_Pin_D13
  Data Store Read11 : DataStoreRead  DataStoreName=Toggle_Pin_D12
  Data Store Read12 : DataStoreRead  DataStoreName=Toggle_Pin_D9
  Data Store Read13 : DataStoreRead  DataStoreName=Toggle_Pin_D8
  Data Store Read14 : DataStoreRead  Priority=71  DataStoreName=Toggle_Pin_D10
  Data Store Read2 : DataStoreRead  Priority=71  DataStoreName=Toggle_Pin_A0
  Data Store Read3 : DataStoreRead  Priority=71  DataStoreName=Toggle_Pin_A1
  Data Store Read4 : DataStoreRead  Priority=21  DataStoreName=Local_Ticks
  Data Store Read5 : DataStoreRead  Priority=81  DataStoreName=Local_Ticks
  Data Store Read6 : DataStoreRead  Priority=80  DataStoreName=Desync_Positive
  Data Store Read7 : DataStoreRead  DataStoreName=basic_cycle_count
  Data Store Read8 : DataStoreRead  Priority=50  DataStoreName=Initialization_flag
  Data Store Read9 : DataStoreRead  DataStoreName=basic_cycle_count
  Equal : RelationalOperator  Priority=23  Operator===  OutDataTypeStr=boolean  RndMeth=Simplest
  Equal1 : RelationalOperator  Priority=23  Operator===  OutDataTypeStr=boolean  RndMeth=Simplest
  Initialization : Subsystem  Priority=8
  LT_Update Desync_Positive : Subsystem  Priority=82  TreatAsAtomicUnit=on
  Logic Analyzer - COMM delay CAN1 - Rx : Subsystem  Priority=74  TreatAsAtomicUnit=on
  Logic Analyzer - COMM delay CAN1 - Tx : Subsystem  Priority=74  TreatAsAtomicUnit=on
  Logic Analyzer - COMM delay CAN2 - Rx : Subsystem  Priority=74  TreatAsAtomicUnit=on
  Logic Analyzer - COMM delay CAN2 - Tx : Subsystem  Priority=74  TreatAsAtomicUnit=on
  Matrix Cycle Manager : Subsystem  Priority=52
  NOT1 : Logic  Priority=51  Operator=NOT  IconShape=distinctive  AllPortsSameDT=off  OutDataTypeStr=boolean
  OR : Logic  Priority=54  Operator=OR  IconShape=distinctive  AllPortsSameDT=off  OutDataTypeStr=boolean
  OR1 : Logic  Priority=55  Operator=OR  IconShape=distinctive  AllPortsSameDT=off  OutDataTypeStr=boolean
  Switch : Switch  Criteria=u2 > Threshold
  MEX : Outport
  Send_New_Msg_CAN1 : Outport  Port=2
  Send_New_Msg_CAN2 : Outport  Port=3
  Receive_New_Msg_CAN1 : Outport  Port=4
  Receive_New_Msg_CAN2 : Outport  Port=5
  wires:
  Matrix Cycle Manager/1(Send_Message_CAN1) -> Chart/1(Condition)
  Data Store Read4/1 -> Equal/1
  Equal/1 -> Basic Cycle Increment/Enable
  NOT1/1 -> Matrix Cycle Manager/Enable
  Data Store Read8/1 -> NOT1/1
  Data Store Read/1 -> Initialization/Enable
  Matrix Cycle Manager/3(Receive_Message_CAN1) -> OR/1
  Chart/1(Trigger_Signal()) -> Send_New_Msg_CAN1/1
  OR/1 -> Chart1/1(Condition)
  Data Store Read1/1 -> OR/2, OR1/1
  Chart1/1(Trigger_Signal()) -> Receive_New_Msg_CAN1/1
  Data Store Read2/1 -> AND/1
  Matrix Cycle Manager/4(Receive_Message_CAN2) -> OR1/2
  Chart2/1(Trigger_Signal()) -> Receive_New_Msg_CAN2/1
  OR1/1 -> Chart2/1(Condition)
  Chart3/1(Trigger_Signal()) -> Send_New_Msg_CAN2/1
  Matrix Cycle Manager/2(Send_Message_CAN2) -> Chart3/1(Condition)
  Chart4/1(Trigger_Signal()) -> MEX/1
  Constant2/1 -> DEBUG - Toggle digital pin A2/Enable
  Constant1/1 -> AND/2
  AND/1 -> DEBUG - Toggle digital pin A0/Enable
  Constant3/1 -> Chart4/1(Condition)
  AND1/1 -> DEBUG - Toggle digital pin A1/Enable
  Constant4/1 -> AND1/2
  Data Store Read3/1 -> AND1/1
  Data Store Read5/1 -> LT_Update Desync_Positive/1(Local Time)
  Data Store Read6/1 -> LT_Update Desync_Positive/Enable
  Data Store Read7/1 -> LT_Update Desync_Positive/2(Bacic_Cycle)
  Switch/1 -> Equal/2
  Constant/1 -> Switch/1
  Constant5/1 -> Switch/3
  Data Store Read9/1 -> Equal1/1
  Constant6/1 -> Equal1/2
  Equal1/1 -> Switch/2
  Constant7/1 -> DEBUG - Toggle digital pin A4/Enable
  Data Store Read11/1 -> AND3/2
  Data Store Read10/1 -> AND2/2
  AND2/1 -> Logic Analyzer - COMM delay CAN1 - Tx/Enable
  AND3/1 -> Logic Analyzer - COMM delay CAN1 - Rx/Enable
  Constant8/1 -> AND5/1, AND4/1, AND3/1, AND2/1
  AND4/1 -> Logic Analyzer - COMM delay CAN2 - Tx/Enable
  Data Store Read13/1 -> AND5/2
  AND5/1 -> Logic Analyzer - COMM delay CAN2 - Rx/Enable
  Data Store Read12/1 -> AND4/2
  Data Store Read14/1 -> AND6/1
  Constant9/1 -> AND6/2
  AND6/1 -> DEBUG - Toggle digital pin D10/Enable

== system HANcoder_E407_TTA_Controller_v4_7/HANcoder STM32 Target - E407-STM32 algorithm/TTA CAN System/CAN1 Recieve/Buffer ready ==
  note: CAN_Rx - Buffer
      | ready for new message
  note: Logic Analyzer - DEBUG
      | Rx Buffer Ready
  Enable : EnablePort
  Data Store Write : DataStoreWrite  DataStoreName=Rx_State_CAN1
  Data Store Write1 : DataStoreWrite  DataStoreName=Toggle_Pin_A0
  New_Msg : Constant  Value=2  OutDataTypeStr=uint8
  SET : Constant  OutDataTypeStr=boolean
  wires:
  New_Msg/1 -> Data Store Write/1
  SET/1 -> Data Store Write1/1

== system HANcoder_E407_TTA_Controller_v4_7/HANcoder STM32 Target - E407-STM32 algorithm/TTA CAN System/CAN1 Recieve/Prepare buffer ==
  note: Start preparing the buffer
  note: Logic Analyzer - DEBUG
      | Preparing Rx buffer
  Enable : EnablePort
  Constant1 : Constant  OutDataTypeStr=uint8
  Data Store Write : DataStoreWrite  DataStoreName=Rx_State_CAN1
  Data Store Write1 : DataStoreWrite  DataStoreName=Toggle_Pin_A0
  SET : Constant  OutDataTypeStr=boolean
  wires:
  Constant1/1 -> Data Store Write/1
  SET/1 -> Data Store Write1/1

== system HANcoder_E407_TTA_Controller_v4_7/HANcoder STM32 Target - E407-STM32 algorithm/TTA CAN System/CAN1 Recieve/RxID_CAN ==
  RxID : Inport
  Bus Creator4 : BusCreator  Inputs=8
  Bus Selector : BusSelector  OutputSignals=signal1,signal2,signal3,signal4,signal5,signal6,signal7,signal8,signal9
  Bus Creator{,1..3,5..9} (9 alike) : BusCreator  Inputs=9
  Constant : Constant  Value=Sync_ID
  Constant1 : Constant  Value=Vote1_ID
  Constant2 : Constant  Value=Vote2_ID
  Constant3 : Constant  Value=Vote3_ID
  Constant4 : Constant  Value=SetValues_ID
  Constant5 : Constant  Value=SensorValues_ID
  Constant6 : Constant  Value=OutControl1_ID
  Constant7 : Constant  Value=OutControl2_ID
  Constant8 : Constant  Value=OutEmulator_ID
  Equal{,1..8} (9 alike) : RelationalOperator  Operator===  OutDataTypeStr=boolean  RndMeth=Simplest
  OutControl1_ID_CAN : Subsystem
  OutControl2_ID_CAN : Subsystem
  OutEmulator_ID_CAN : Subsystem
  SensorValues_ID_CAN : Subsystem
  SetValues_ID_CAN : Subsystem
  Switch{,1..7} (8 alike) : Switch  Criteria=u2 > Threshold
  Sync_ID_CAN : Subsystem
  Vote1_ID_CAN : Subsystem
  Vote2_ID_CAN : Subsystem
  Vote3_ID_CAN : Subsystem
  CAN_new : Outport
  message : Outport  Port=2
  wires:
  Constant/1 -> Equal/2
  Equal/1 -> Sync_ID_CAN/Enable, Switch/2
  Constant1/1 -> Equal1/2
  Constant2/1 -> Equal2/2
  Constant3/1 -> Equal3/2
  Equal1/1 -> Vote1_ID_CAN/Enable, Switch1/2
  Equal2/1 -> Vote2_ID_CAN/Enable, Switch2/2
  Equal3/1 -> Vote3_ID_CAN/Enable, Switch3/2
  Sync_ID_CAN/1(CAN_new) -> Bus Creator/1
  Sync_ID_CAN/2(Out2) -> Bus Creator/2
  Sync_ID_CAN/3(Out3) -> Bus Creator/3
  Sync_ID_CAN/4(Out4) -> Bus Creator/4
  Sync_ID_CAN/5(Out5) -> Bus Creator/5
  Sync_ID_CAN/6(Out6) -> Bus Creator/6
  Sync_ID_CAN/7(Out7) -> Bus Creator/7
  Sync_ID_CAN/8(Out8) -> Bus Creator/8
  Sync_ID_CAN/9(Out9) -> Bus Creator/9
  Bus Creator/1 -> Switch/1
  Vote1_ID_CAN/1(CAN_new) -> Bus Creator1/1
  Vote1_ID_CAN/2(Out2) -> Bus Creator1/2
  Vote1_ID_CAN/3(Out3) -> Bus Creator1/3
  Vote1_ID_CAN/4(Out4) -> Bus Creator1/4
  Vote1_ID_CAN/5(Out5) -> Bus Creator1/5
  Vote1_ID_CAN/6(Out6) -> Bus Creator1/6
  Vote1_ID_CAN/7(Out7) -> Bus Creator1/7
  Vote1_ID_CAN/8(Out8) -> Bus Creator1/8
  Vote1_ID_CAN/9(Out9) -> Bus Creator1/9
  Bus Creator1/1 -> Switch1/1
  Vote2_ID_CAN/1(CAN_new) -> Bus Creator2/1
  Vote2_ID_CAN/2(Out2) -> Bus Creator2/2
  Vote2_ID_CAN/3(Out3) -> Bus Creator2/3
  Vote2_ID_CAN/4(Out4) -> Bus Creator2/4
  Vote2_ID_CAN/6(Out6) -> Bus Creator2/6
  Vote2_ID_CAN/5(Out5) -> Bus Creator2/5
  Vote2_ID_CAN/7(Out7) -> Bus Creator2/7
  Vote2_ID_CAN/8(Out8) -> Bus Creator2/8
  Vote2_ID_CAN/9(Out9) -> Bus Creator2/9
  Bus Creator2/1 -> Switch2/1
  Vote3_ID_CAN/1(CAN_new) -> Bus Creator3/1
  Vote3_ID_CAN/2(Out2) -> Bus Creator3/2
  Vote3_ID_CAN/3(Out3) -> Bus Creator3/3
  Vote3_ID_CAN/4(Out4) -> Bus Creator3/4
  Vote3_ID_CAN/5(Out5) -> Bus Creator3/5
  Vote3_ID_CAN/6(Out6) -> Bus Creator3/6
  Vote3_ID_CAN/7(Out7) -> Bus Creator3/7
  Vote3_ID_CAN/8(Out8) -> Bus Creator3/8
  Vote3_ID_CAN/9(Out9) -> Bus Creator3/9
  Bus Creator3/1 -> Switch3/1
  Switch1/1 -> Switch/3
  Switch2/1 -> Switch1/3
  Switch/1 -> Bus Selector/1
  Bus Selector/1 -> CAN_new/1  "<signal1>"
  Bus Creator4/1 -> message/1
  Bus Selector/2 -> Bus Creator4/1  "<signal2>"
  Bus Selector/6 -> Bus Creator4/5  "<signal6>"
  Bus Selector/7 -> Bus Creator4/6  "<signal7>"
  Bus Selector/8 -> Bus Creator4/7  "<signal8>"
  Bus Selector/9 -> Bus Creator4/8  "<signal9>"
  Bus Selector/3 -> Bus Creator4/2  "<signal3>"
  Bus Selector/4 -> Bus Creator4/3  "<signal4>"
  Bus Selector/5 -> Bus Creator4/4  "<signal5>"
  Switch3/1 -> Switch2/3
  Switch4/1 -> Switch3/3
  Switch5/1 -> Switch4/3
  SetValues_ID_CAN/9(Out9) -> Bus Creator5/9
  SetValues_ID_CAN/8(Out8) -> Bus Creator5/8
  SetValues_ID_CAN/7(Out7) -> Bus Creator5/7
  SetValues_ID_CAN/6(Out6) -> Bus Creator5/6
  SetValues_ID_CAN/5(Out5) -> Bus Creator5/5
  SetValues_ID_CAN/2(Out2) -> Bus Creator5/2
  SetValues_ID_CAN/1(CAN_new) -> Bus Creator5/1
  SetValues_ID_CAN/3(Out3) -> Bus Creator5/3
  SetValues_ID_CAN/4(Out4) -> Bus Creator5/4
  Bus Creator5/1 -> Switch4/1
  Constant4/1 -> Equal4/2
  Equal4/1 -> SetValues_ID_CAN/Enable, Switch4/2
  Equal5/1 -> Switch5/2, SensorValues_ID_CAN/Enable
  Constant5/1 -> Equal5/2
  Bus Creator6/1 -> Switch5/1
  SensorValues_ID_CAN/4(Out4) -> Bus Creator6/4
  SensorValues_ID_CAN/3(Out3) -> Bus Creator6/3
  SensorValues_ID_CAN/1(CAN_new) -> Bus Creator6/1
  SensorValues_ID_CAN/2(Out2) -> Bus Creator6/2
  SensorValues_ID_CAN/5(Out5) -> Bus Creator6/5
  SensorValues_ID_CAN/6(Out6) -> Bus Creator6/6
  SensorValues_ID_CAN/7(Out7) -> Bus Creator6/7
  SensorValues_ID_CAN/8(Out8) -> Bus Creator6/8
  SensorValues_ID_CAN/9(Out9) -> Bus Creator6/9
  OutControl1_ID_CAN/9(Out9) -> Bus Creator7/9
  OutControl1_ID_CAN/8(Out8) -> Bus Creator7/8
  OutControl1_ID_CAN/7(Out7) -> Bus Creator7/7
  OutControl1_ID_CAN/6(Out6) -> Bus Creator7/6
  OutControl1_ID_CAN/5(Out5) -> Bus Creator7/5
  OutControl1_ID_CAN/2(Out2) -> Bus Creator7/2
  OutControl1_ID_CAN/1(CAN_new) -> Bus Creator7/1
  OutControl1_ID_CAN/3(Out3) -> Bus Creator7/3
  OutControl1_ID_CAN/4(Out4) -> Bus Creator7/4
  Constant6/1 -> Equal6/2
  Equal6/1 -> Switch6/2, OutControl1_ID_CAN/Enable
  Bus Creator7/1 -> Switch6/1
  Bus Creator8/1 -> Switch7/1
  Equal7/1 -> Switch7/2, OutControl2_ID_CAN/Enable
  Constant7/1 -> Equal7/2
  OutControl2_ID_CAN/4(Out4) -> Bus Creator8/4
  OutControl2_ID_CAN/3(Out3) -> Bus Creator8/3
  OutControl2_ID_CAN/1(CAN_new) -> Bus Creator8/1
  OutControl2_ID_CAN/2(Out2) -> Bus Creator8/2
  OutControl2_ID_CAN/5(Out5) -> Bus Creator8/5
  OutControl2_ID_CAN/6(Out6) -> Bus Creator8/6
  OutControl2_ID_CAN/7(Out7) -> Bus Creator8/7
  OutControl2_ID_CAN/8(Out8) -> Bus Creator8/8
  OutControl2_ID_CAN/9(Out9) -> Bus Creator8/9
  OutEmulator_ID_CAN/9(Out9) -> Bus Creator9/9
  OutEmulator_ID_CAN/8(Out8) -> Bus Creator9/8
  OutEmulator_ID_CAN/7(Out7) -> Bus Creator9/7
  OutEmulator_ID_CAN/6(Out6) -> Bus Creator9/6
  OutEmulator_ID_CAN/5(Out5) -> Bus Creator9/5
  OutEmulator_ID_CAN/2(Out2) -> Bus Creator9/2
  OutEmulator_ID_CAN/1(CAN_new) -> Bus Creator9/1
  OutEmulator_ID_CAN/3(Out3) -> Bus Creator9/3
  OutEmulator_ID_CAN/4(Out4) -> Bus Creator9/4
  Constant8/1 -> Equal8/2
  RxID/1 -> Equal2/1, Equal6/1, Equal7/1, Equal8/1, Equal5/1, Equal4/1, Equal3/1, Equal1/1, Equal/1
  Equal8/1 -> OutEmulator_ID_CAN/Enable
  Bus Creator9/1 -> Switch7/3
  Switch7/1 -> Switch6/3
  Switch6/1 -> Switch5/3
